simulink model "pcopy_offline_test"  (R2017a)
settings: Solver=VariableStepAuto  StartTime=0.0  StopTime=20  RelTol=1e-3
settings Model: Creator=Administrator  LastModifiedBy=Administrator
settings OptimizationCC: LifeSpan=inf
settings DebuggingCC: SFExecutionAtInitializationDiag=none

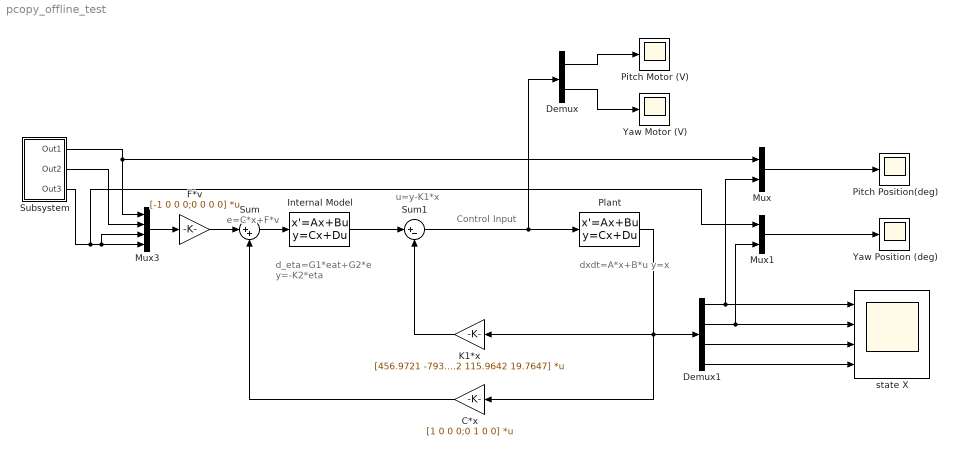
== system pcopy_offline_test ==
  note: Control Input
  note: e=C*x+F*v
  note: dxdt=A*x+B*u
      |      y=x
  note: d_eta=G1*eat+G2*e
      |        y=-K2*eta
  note: u=y-K1*x
  C*x : Gain  Gain=[1 0 0 0;0 1 0 0]  Multiplication=Matrix(K*u)
  Demux : Demux  Outputs=2
  Demux1 : Demux
  F*v : Gain  Gain=[-1 0 0 0;0 0 0 0]  Multiplication=Matrix(K*u)
  Internal Model : StateSpace  A=[0 1 0 0 0 0;0 0 1 0 0 0;0 -1 0 0 0 0;0 0 0 0 1 0;0 0 0 0 0 1;0 0 0 0 -1 0]  B=[0 0;0 0;1 0;0 0;0 0;0 1]  C=[-139.1 -1888 -1334.1 5664.7 5615 3110.8;-4892.1 -5540.6 -3198.1 2116.5 577.4 57.8]  D=[0 0;0 0]  X0=[1 0 2 1 0 2]
  K1*x : Gain  Gain=[456.9721 -793.3427 70.3033 -98.0538;856.0024 97.9162 115.9642 19.7647]  Multiplication=Matrix(K*u)
  Mux : Mux  Inputs=2
  Mux1 : Mux  Inputs=2
  Mux3 : Mux
  Pitch Motor (V) : Scope
  Pitch Position(deg) : Scope
  Plant : StateSpace  A=[0 0 1 0;0 0 0 1;-1.7117 0 -0.3249 0;0 0 0 -1.0004]  B=[0 0;0 0;0.0503 0.0959;-0.1228 0.1]  C=[1 0 0 0;0 1 0 0;0 0 1 0;0 0 0 1]  D=[0 0;0 0;0 0;0 0]  X0=[2 1 0 0]
  Subsystem : Subsystem
  Sum : Sum  Inputs=|++
  Sum1 : Sum  Inputs=|+-
  Yaw Motor (V) : Scope
  Yaw Position (deg) : Scope
  state X : Scope  NumInputPorts=4
  wires:
  Subsystem/1(Out1) -> Mux/1, Mux3/1
  Subsystem/3(Out3) -> Mux1/1, Mux3/3, Mux3/4
  Demux1/3 -> state X/3
  Internal Model/1 -> Sum1/1
  F*v/1 -> Sum/1
  Plant/1 -> C*x/1, Demux1/1, K1*x/1
  Demux1/1 -> state X/1, Mux/2
  Demux/2 -> Yaw Motor (V)/1
  Sum/1 -> Internal Model/1
  Mux3/1 -> F*v/1
  C*x/1 -> Sum/2
  Subsystem/2(Out2) -> Mux3/2
  Mux/1 -> Pitch Position(deg)/1
  Demux1/4 -> state X/4
  Sum1/1 -> Plant/1, Demux/1
  Mux1/1 -> Yaw Position (deg)/1
  K1*x/1 -> Sum1/2
  Demux/1 -> Pitch Motor (V)/1
  Demux1/2 -> state X/2, Mux1/2

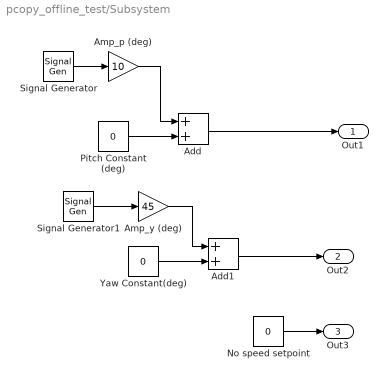
== system pcopy_offline_test/Subsystem ==
  Add : Sum
  Add1 : Sum
  Amp_p (deg) : Gain  Gain=10
  Amp_y (deg) : Gain  Gain=45
  No speed setpoint : Constant  Value=0
  Pitch Constant (deg) : Constant  Value=0
  Signal Generator : SignalGenerator  Frequency=0.1
  Signal Generator1 : SignalGenerator  Frequency=0.04
  Yaw Constant(deg) : Constant  Value=0
  Out1 : Outport
  Out2 : Outport  Port=2
  Out3 : Outport  Port=3
  wires:
  Pitch Constant (deg)/1 -> Add/2
  Signal Generator/1 -> Amp_p (deg)/1
  Add1/1 -> Out2/1
  Add/1 -> Out1/1
  Signal Generator1/1 -> Amp_y (deg)/1
  Amp_y (deg)/1 -> Add1/1
  Yaw Constant(deg)/1 -> Add1/2
  Amp_p (deg)/1 -> Add/1
  No speed setpoint/1 -> Out3/1
